simulink model "M_DYN_AerodynamicData"  (R2022a)
settings: Solver=ode4  StartTime=0.0  StopTime=0.04  FixedStep=0.01  RelTol=1e-3
PreLoadFcn:
  | load('f16data.mat');
InitFcn:
  | load('f16data.mat');
values from neighbouring files (symbols this model uses):
  f16data =     [f16data.mat]
settings Model: Creator=ASCL  LastModifiedBy=ASCL
settings DataIOCC: SaveOutput=off  SignalLogging=off  DSMLogging=off  SaveTime=off  ReturnWorkspaceOutputs=off
settings OptimizationCC: BlockReduction=off  DefaultParameterBehavior=Inlined  UseDivisionForNetSlopeComputation=on  GainParamInheritBuiltInType=on  UseFloatMulNetSlope=on  ExpressionFolding=off  PassReuseOutputArgsAs=Individual arguments  ZeroExternalMemoryAtStartup=off  ZeroInternalMemoryAtStartup=off  EfficientFloat2IntCast=on  LifeSpan=inf  OptimizeBlockOrder=speed  DifferentSizesBufferReuse=on  EfficientTunableParamExpr=on
settings DebuggingCC: SignalInfNanChecking=warning  ReadBeforeWriteMsg=EnableAllAsError  WriteAfterWriteMsg=EnableAllAsError  WriteAfterReadMsg=EnableAllAsError  IntegerOverflowMsg=error  ParameterTunabilityLossMsg=error  UniqueDataStoreMsg=error  AssertControl=DisableAll  NonBusSignalsTreatedAsBus=error  SFInvalidInputDataAccessInChartInitDiag=error  SFTransitionOutsideNaturalParentDiag=error  SFUnreachableExecutionPathDiag=error  SFUndirectedBroadcastEventsDiag=error  IntegerSaturationMsg=error
settings HardwareCC: ProdBitPerPointer=32  ProdBitPerSizeT=32  ProdBitPerPtrDiffT=32  ProdLargestAtomicInteger=Long  ProdLargestAtomicFloat=Double  ProdEndianess=BigEndian  ProdWordSize=32  ProdLongLongMode=on  ProdHWDeviceType=Freescale->MPC83xx
settings SFSimCC: CompileTimeRecursionLimit=0  EnableRuntimeRecursion=off  MATLABDynamicMemAlloc=off
settings RTWCC: SystemTargetFile=ert.tlc  TemplateMakefile=ert_default_tmf  GenerateReport=on  RTWUseSimCustomCode=on  BuildConfiguration=Faster Runs  IncludeHyperlinkInReport=on  LaunchReport=on  GenerateTraceInfo=on  GenerateTraceReport=on  GenerateTraceReportSl=on  GenerateTraceReportSf=on  GenerateTraceReportEml=on
settings CodeAppCC: ForceParamTrailComments=on  IgnoreCustomStorageClasses=off  OperatorAnnotations=on  SimulinkDataObjDesc=on  SFDataObjDesc=on  MATLABFcnDesc=on  InsertBlockDesc=on  StateflowObjectComments=on  MATLABSourceComments=on  EnableCustomComments=on  InlinedPrmAccess=Macros  ReqsInCode=on
settings ERTTargetCC: TargetLangStandard=C99 (ISO)  UtilityFuncGeneration=Shared location  GenerateSampleERTMain=on  IncludeMdlTerminateFcn=off  CombineSignalStateStructs=on  SupportAbsoluteTime=off  SupportNonFinite=off  SupportVariableSizeSignals=on  ParenthesesLevel=Standards  CastingMode=Standards  GenerateSharedConstants=off  InlinedParameterPlacement=NonHierarchical  ERTCustomFileTemplate=example_file_process.tlc  RateTransitionBlockCode=Function  PreserveIfCondition=on  ConvertIfToSwitch=off  EnableSignedLeftShifts=off  EnableSignedRightShifts=off

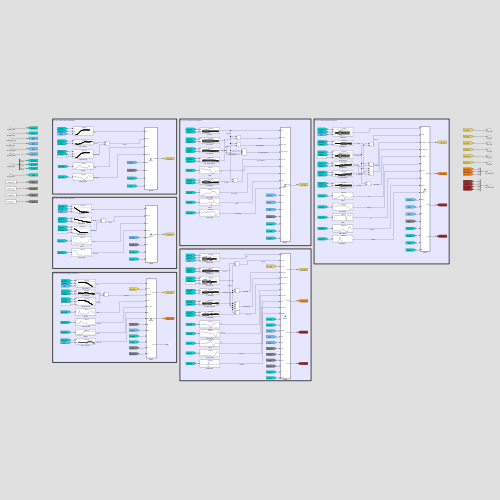
[thumbnail: Simulink's stored preview of the top-level diagram]
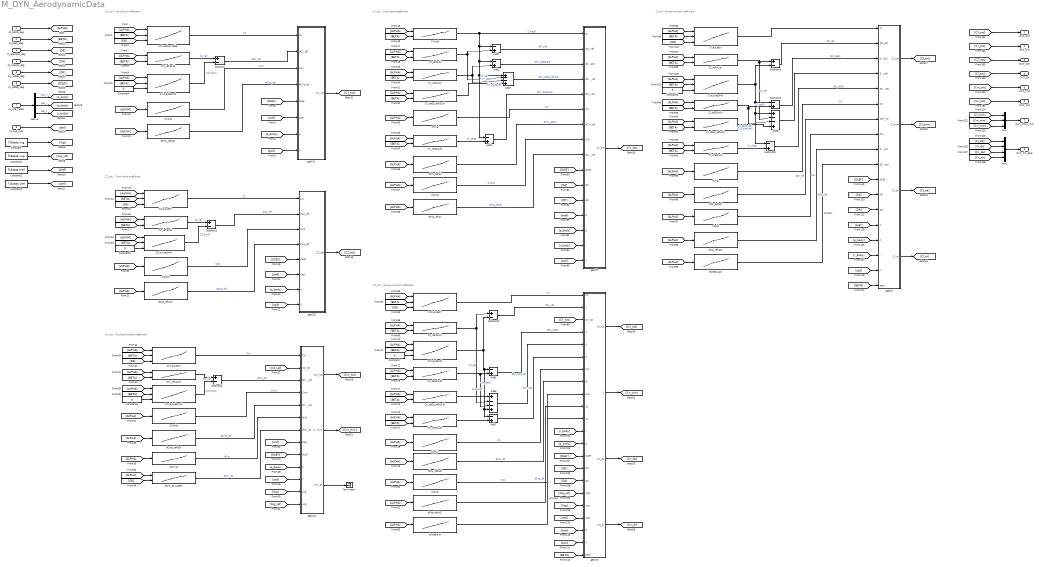
== system M_DYN_AerodynamicData ==
  note: Cl_tot : rolling moment coefficient
  note: Cn_tot : yawing moment coefficient
  note: CY_tot : Y-axis force coefficient
  note: Cm_tot : Pitching moment coefficient
  note: CZ_tot : Z-axis force coefficient
  note: CX_tot: X-axis force coefficient
  IN_alpha_deg : Inport  Interpolate=off
  IN_beta_deg : Inport  Port=2  Interpolate=off
  IN_elevator_deg : Inport  Port=3  Interpolate=off
  IN_aileron_deg : Inport  Port=4  Interpolate=off
  IN_rudder_deg : Inport  Port=5  Interpolate=off
  IN_LEflap_deg : Inport  Port=6  Interpolate=off
  IN_WB_radps : Inport  Port=7  Interpolate=off
  IN_spd_mps : Inport  Port=8  Interpolate=off
  Add{1..2,4..5,7} (5 alike) : Sum  Inputs=-+
  Add3 : Sum  Inputs=+--+
  Add6 : Sum  Inputs=+--+
  Add8 : Sum  Inputs=+--+
  CX(a,b,de1=0) : Lookup_n-D  NumberOfTableDimensions=3  BreakpointsForDimension1=f16data.alpha1  BreakpointsForDimension2=f16data.beta  BreakpointsForDimension3=f16data.de1  Table=f16data.CX  InternalRulePriority=Speed  RndMeth=Simplest
      settings: InputPortMap=u0,u1,u2
  CX_lef(a2,b) : Lookup_n-D  LookupTableObject=''  BreakpointsForDimension1=f16data.alpha2  BreakpointsForDimension2=f16data.beta  BreakpointsForDimension1FirstPoint=10  BreakpointsForDimension2FirstPoint=10  BreakpointsForDimension1Spacing=12  BreakpointsForDimension2Spacing=12  Table=f16data.CX_lef  DiagnosticForOutOfRangeInput=Warning  InternalRulePriority=Speed  RndMeth=Simplest
      settings: InputPortMap=u0,u1
  CXq(a) : Lookup_n-D  NumberOfTableDimensions=1  BreakpointsForDimension1=f16data.alpha1  Table=f16data.CXq  InternalRulePriority=Speed  RndMeth=Simplest
  CY(a,b) : Lookup_n-D  LookupTableObject=''  BreakpointsForDimension1=f16data.alpha1  BreakpointsForDimension2=f16data.beta  BreakpointsForDimension1FirstPoint=10  BreakpointsForDimension2FirstPoint=10  BreakpointsForDimension1Spacing=12  BreakpointsForDimension2Spacing=12  Table=f16data.CY  DiagnosticForOutOfRangeInput=Warning  InternalRulePriority=Speed  RndMeth=Simplest
      settings: InputPortMap=u0,u1
  CY_a20(a,b) : Lookup_n-D  LookupTableObject=''  BreakpointsForDimension1=f16data.alpha1  BreakpointsForDimension2=f16data.beta  BreakpointsForDimension1FirstPoint=10  BreakpointsForDimension2FirstPoint=10  BreakpointsForDimension1Spacing=12  BreakpointsForDimension2Spacing=12  Table=f16data.CY_da20  DiagnosticForOutOfRangeInput=Warning  InternalRulePriority=Speed  RndMeth=Simplest
      settings: InputPortMap=u0,u1
  CY_da20_lef(a2,b) : Lookup_n-D  LookupTableObject=''  BreakpointsForDimension1=f16data.alpha2  BreakpointsForDimension2=f16data.beta  BreakpointsForDimension1FirstPoint=10  BreakpointsForDimension2FirstPoint=10  BreakpointsForDimension1Spacing=12  BreakpointsForDimension2Spacing=12  Table=f16data.CY_da20lef  DiagnosticForOutOfRangeInput=Warning  InternalRulePriority=Speed  RndMeth=Simplest
      settings: InputPortMap=u0,u1
  CY_dr30(a,b) : Lookup_n-D  LookupTableObject=''  BreakpointsForDimension1=f16data.alpha1  BreakpointsForDimension2=f16data.beta  BreakpointsForDimension1FirstPoint=10  BreakpointsForDimension2FirstPoint=10  BreakpointsForDimension1Spacing=12  BreakpointsForDimension2Spacing=12  Table=f16data.CY_dr30  DiagnosticForOutOfRangeInput=Warning  InternalRulePriority=Speed  RndMeth=Simplest
      settings: InputPortMap=u0,u1
  CY_lef(a,b) : Lookup_n-D  LookupTableObject=''  BreakpointsForDimension1=f16data.alpha2  BreakpointsForDimension2=f16data.beta  BreakpointsForDimension1FirstPoint=10  BreakpointsForDimension2FirstPoint=10  BreakpointsForDimension1Spacing=12  BreakpointsForDimension2Spacing=12  Table=f16data.CY_lef  DiagnosticForOutOfRangeInput=Warning  InternalRulePriority=Speed  RndMeth=Simplest
      settings: InputPortMap=u0,u1
  CYp(a) : Lookup_n-D  NumberOfTableDimensions=1  LookupTableObject=''  BreakpointsForDimension1=f16data.alpha1  BreakpointsForDimension2=f16data.beta  BreakpointsForDimension1FirstPoint=10  BreakpointsForDimension2FirstPoint=10  BreakpointsForDimension1Spacing=12  BreakpointsForDimension2Spacing=12  Table=f16data.CYp  DiagnosticForOutOfRangeInput=Warning  InternalRulePriority=Speed  RndMeth=Simplest
  CYr(a) : Lookup_n-D  NumberOfTableDimensions=1  LookupTableObject=''  BreakpointsForDimension1=f16data.alpha1  BreakpointsForDimension2=f16data.beta  BreakpointsForDimension1FirstPoint=10  BreakpointsForDimension2FirstPoint=10  BreakpointsForDimension1Spacing=12  BreakpointsForDimension2Spacing=12  Table=f16data.CYr  DiagnosticForOutOfRangeInput=Warning  InternalRulePriority=Speed  RndMeth=Simplest
  CZ(a,b,de1) : Lookup_n-D  NumberOfTableDimensions=3  BreakpointsForDimension1=f16data.alpha1  BreakpointsForDimension2=f16data.beta  BreakpointsForDimension3=f16data.de1  BeginIndexSearchUsingPreviousIndexResult=on  Table=f16data.CZ  InternalRulePriority=Speed  RndMeth=Simplest
      settings: InputPortMap=u0,u1,u2
  CZ(a,b,de1=0) : Lookup_n-D  NumberOfTableDimensions=3  BreakpointsForDimension1=f16data.alpha1  BreakpointsForDimension2=f16data.beta  BreakpointsForDimension3=f16data.de1  BeginIndexSearchUsingPreviousIndexResult=on  Table=f16data.CZ  InternalRulePriority=Speed  RndMeth=Simplest
      settings: InputPortMap=u0,u1,u2
  CZ_lef(a2,b) : Lookup_n-D  LookupTableObject=''  BreakpointsForDimension1=f16data.alpha2  BreakpointsForDimension2=f16data.beta  BreakpointsForDimension1FirstPoint=10  BreakpointsForDimension2FirstPoint=10  BreakpointsForDimension1Spacing=12  BreakpointsForDimension2Spacing=12  BeginIndexSearchUsingPreviousIndexResult=on  Table=f16data.CZ_lef  DiagnosticForOutOfRangeInput=Warning  InternalRulePriority=Speed  RndMeth=Simplest
      settings: InputPortMap=u0,u1
  CZq(a) : Lookup_n-D  NumberOfTableDimensions=1  BreakpointsForDimension1=f16data.alpha1  BeginIndexSearchUsingPreviousIndexResult=on  Table=f16data.CZq  InternalRulePriority=Speed  RndMeth=Simplest
  Cl(a,b,de2) : Lookup_n-D  NumberOfTableDimensions=3  BreakpointsForDimension1=f16data.alpha1  BreakpointsForDimension2=f16data.beta  BreakpointsForDimension3=f16data.de2  Table=f16data.Cl  InternalRulePriority=Speed  RndMeth=Simplest
      settings: InputPortMap=u0,u1,u2
  Cl(a,b,de2=0) : Lookup_n-D  NumberOfTableDimensions=3  BreakpointsForDimension1=f16data.alpha1  BreakpointsForDimension2=f16data.beta  BreakpointsForDimension3=f16data.de2  Table=f16data.Cl  InternalRulePriority=Speed  RndMeth=Simplest
      settings: InputPortMap=u0,u1,u2
  Cl_da20(a,b) : Lookup_n-D  LookupTableObject=''  BreakpointsForDimension1=f16data.alpha1  BreakpointsForDimension2=f16data.beta  BreakpointsForDimension1FirstPoint=10  BreakpointsForDimension2FirstPoint=10  BreakpointsForDimension1Spacing=12  BreakpointsForDimension2Spacing=12  Table=f16data.Cl_da20  DiagnosticForOutOfRangeInput=Warning  InternalRulePriority=Speed  RndMeth=Simplest
      settings: InputPortMap=u0,u1
  Cl_da20_lef(a,b) : Lookup_n-D  LookupTableObject=''  BreakpointsForDimension1=f16data.alpha2  BreakpointsForDimension2=f16data.beta  BreakpointsForDimension1FirstPoint=10  BreakpointsForDimension2FirstPoint=10  BreakpointsForDimension1Spacing=12  BreakpointsForDimension2Spacing=12  Table=f16data.Cl_da20lef  DiagnosticForOutOfRangeInput=Warning  InternalRulePriority=Speed  RndMeth=Simplest
      settings: InputPortMap=u0,u1
  Cl_dr30(a,b) : Lookup_n-D  LookupTableObject=''  BreakpointsForDimension1=f16data.alpha1  BreakpointsForDimension2=f16data.beta  BreakpointsForDimension1FirstPoint=10  BreakpointsForDimension2FirstPoint=10  BreakpointsForDimension1Spacing=12  BreakpointsForDimension2Spacing=12  Table=f16data.Cl_dr30  DiagnosticForOutOfRangeInput=Warning  InternalRulePriority=Speed  RndMeth=Simplest
      settings: InputPortMap=u0,u1
  Cl_lef(a2,b) : Lookup_n-D  LookupTableObject=''  BreakpointsForDimension1=f16data.alpha2  BreakpointsForDimension2=f16data.beta  BreakpointsForDimension1FirstPoint=10  BreakpointsForDimension2FirstPoint=10  BreakpointsForDimension1Spacing=12  BreakpointsForDimension2Spacing=12  Table=f16data.Cl_lef  DiagnosticForOutOfRangeInput=Warning  InternalRulePriority=Speed  RndMeth=Simplest
      settings: InputPortMap=u0,u1
  Clp(a) : Lookup_n-D  NumberOfTableDimensions=1  LookupTableObject=''  BreakpointsForDimension1=f16data.alpha1  BreakpointsForDimension2=f16data.beta  BreakpointsForDimension1FirstPoint=10  BreakpointsForDimension2FirstPoint=10  BreakpointsForDimension1Spacing=12  BreakpointsForDimension2Spacing=12  Table=f16data.Clp  DiagnosticForOutOfRangeInput=Warning  InternalRulePriority=Speed  RndMeth=Simplest
  Clr(a) : Lookup_n-D  NumberOfTableDimensions=1  LookupTableObject=''  BreakpointsForDimension1=f16data.alpha1  BreakpointsForDimension2=f16data.beta  BreakpointsForDimension1FirstPoint=10  BreakpointsForDimension2FirstPoint=10  BreakpointsForDimension1Spacing=12  BreakpointsForDimension2Spacing=12  Table=f16data.Clr  DiagnosticForOutOfRangeInput=Warning  InternalRulePriority=Speed  RndMeth=Simplest
  Cm(a,b,de1) : Lookup_n-D  NumberOfTableDimensions=3  BreakpointsForDimension1=f16data.alpha1  BreakpointsForDimension2=f16data.beta  BreakpointsForDimension3=f16data.de1  Table=f16data.Cm  InternalRulePriority=Speed  RndMeth=Simplest
      settings: InputPortMap=u0,u1,u2
  Cm(a,b,de1=0) : Lookup_n-D  NumberOfTableDimensions=3  BreakpointsForDimension1=f16data.alpha1  BreakpointsForDimension2=f16data.beta  BreakpointsForDimension3=f16data.de1  Table=f16data.Cm  InternalRulePriority=Speed  RndMeth=Simplest
      settings: InputPortMap=u0,u1,u2
  Cm_lef(a2,b) : Lookup_n-D  LookupTableObject=''  BreakpointsForDimension1=f16data.alpha2  BreakpointsForDimension2=f16data.beta  BreakpointsForDimension1FirstPoint=10  BreakpointsForDimension2FirstPoint=10  BreakpointsForDimension1Spacing=12  BreakpointsForDimension2Spacing=12  Table=f16data.Cm_lef  DiagnosticForOutOfRangeInput=Warning  InternalRulePriority=Speed  RndMeth=Simplest
      settings: InputPortMap=u0,u1
  Cmq(a) : Lookup_n-D  NumberOfTableDimensions=1  BreakpointsForDimension1=f16data.alpha1  Table=f16data.Cmq  InternalRulePriority=Speed  RndMeth=Simplest
  Cn(a,b,de2) : Lookup_n-D  NumberOfTableDimensions=3  BreakpointsForDimension1=f16data.alpha1  BreakpointsForDimension2=f16data.beta  BreakpointsForDimension3=f16data.de2  Table=f16data.Cn  InternalRulePriority=Speed  RndMeth=Simplest
      settings: InputPortMap=u0,u1,u2
  Cn(a,b,de=0) : Lookup_n-D  NumberOfTableDimensions=3  BreakpointsForDimension1=f16data.alpha1  BreakpointsForDimension2=f16data.beta  BreakpointsForDimension3=f16data.de2  Table=f16data.Cn  InternalRulePriority=Speed  RndMeth=Simplest
      settings: InputPortMap=u0,u1,u2
  Cn_da20(a,b) : Lookup_n-D  LookupTableObject=''  BreakpointsForDimension1=f16data.alpha1  BreakpointsForDimension2=f16data.beta  BreakpointsForDimension1FirstPoint=10  BreakpointsForDimension2FirstPoint=10  BreakpointsForDimension1Spacing=12  BreakpointsForDimension2Spacing=12  Table=f16data.Cn_da20  DiagnosticForOutOfRangeInput=Warning  InternalRulePriority=Speed  RndMeth=Simplest
      settings: InputPortMap=u0,u1
  Cn_da20_lef(a2,b) : Lookup_n-D  LookupTableObject=''  BreakpointsForDimension1=f16data.alpha2  BreakpointsForDimension2=f16data.beta  BreakpointsForDimension1FirstPoint=10  BreakpointsForDimension2FirstPoint=10  BreakpointsForDimension1Spacing=12  BreakpointsForDimension2Spacing=12  Table=f16data.Cn_da20lef  DiagnosticForOutOfRangeInput=Warning  InternalRulePriority=Speed  RndMeth=Simplest
      settings: InputPortMap=u0,u1
  Cn_dr30(a,b) : Lookup_n-D  LookupTableObject=''  BreakpointsForDimension1=f16data.alpha1  BreakpointsForDimension2=f16data.beta  BreakpointsForDimension1FirstPoint=10  BreakpointsForDimension2FirstPoint=10  BreakpointsForDimension1Spacing=12  BreakpointsForDimension2Spacing=12  Table=f16data.Cn_dr30  DiagnosticForOutOfRangeInput=Warning  InternalRulePriority=Speed  RndMeth=Simplest
      settings: InputPortMap=u0,u1
  Cn_lef(a2,b) : Lookup_n-D  LookupTableObject=''  BreakpointsForDimension1=f16data.alpha2  BreakpointsForDimension2=f16data.beta  BreakpointsForDimension1FirstPoint=10  BreakpointsForDimension2FirstPoint=10  BreakpointsForDimension1Spacing=12  BreakpointsForDimension2Spacing=12  Table=f16data.Cn_lef  DiagnosticForOutOfRangeInput=Warning  InternalRulePriority=Speed  RndMeth=Simplest
      settings: InputPortMap=u0,u1
  Cnp(a) : Lookup_n-D  NumberOfTableDimensions=1  LookupTableObject=''  BreakpointsForDimension1=f16data.alpha1  BreakpointsForDimension2=f16data.beta  BreakpointsForDimension1FirstPoint=10  BreakpointsForDimension2FirstPoint=10  BreakpointsForDimension1Spacing=12  BreakpointsForDimension2Spacing=12  Table=f16data.Cnp  DiagnosticForOutOfRangeInput=Warning  InternalRulePriority=Speed  RndMeth=Simplest
  Cnr(a) : Lookup_n-D  NumberOfTableDimensions=1  LookupTableObject=''  BreakpointsForDimension1=f16data.alpha1  BreakpointsForDimension2=f16data.beta  BreakpointsForDimension1FirstPoint=10  BreakpointsForDimension2FirstPoint=10  BreakpointsForDimension1Spacing=12  BreakpointsForDimension2Spacing=12  Table=f16data.Cnr  DiagnosticForOutOfRangeInput=Warning  InternalRulePriority=Speed  RndMeth=Simplest
  Constant : Constant  Value=f16data.xcg
  Constant1 : Constant  Value=f16data.xcgr
  Constant2 : Constant  Value=f16data.bref
  Constant3 : Constant  Value=f16data.cref
  Constant{4..8} (5 alike) : Constant  Value=0
  Demux : Demux  Outputs=3
  Mux : Mux  Inputs=3
  Mux1 : Mux
  Subtract{,1..4} (5 alike) : Sum  Inputs=+-
  Subtract5 : Sum  Inputs=-+
  Subtract6 : Sum  Inputs=-+
  Terminator : Terminator
  dCXq_lef(a2) : Lookup_n-D  NumberOfTableDimensions=1  BreakpointsForDimension1=f16data.alpha2  Table=f16data.dCXq_lef  InternalRulePriority=Speed  RndMeth=Simplest
  dCYp_lef(a) : Lookup_n-D  NumberOfTableDimensions=1  LookupTableObject=''  BreakpointsForDimension1=f16data.alpha2  BreakpointsForDimension2=f16data.beta  BreakpointsForDimension1FirstPoint=10  BreakpointsForDimension2FirstPoint=10  BreakpointsForDimension1Spacing=12  BreakpointsForDimension2Spacing=12  Table=f16data.dCYp_lef  DiagnosticForOutOfRangeInput=Warning  InternalRulePriority=Speed  RndMeth=Simplest
  dCYr_lef(a) : Lookup_n-D  NumberOfTableDimensions=1  LookupTableObject=''  BreakpointsForDimension1=f16data.alpha2  BreakpointsForDimension2=f16data.beta  BreakpointsForDimension1FirstPoint=10  BreakpointsForDimension2FirstPoint=10  BreakpointsForDimension1Spacing=12  BreakpointsForDimension2Spacing=12  Table=f16data.dCYr_lef  DiagnosticForOutOfRangeInput=Warning  InternalRulePriority=Speed  RndMeth=Simplest
  dCZq_lef(a2) : Lookup_n-D  NumberOfTableDimensions=1  BreakpointsForDimension1=f16data.alpha2  BeginIndexSearchUsingPreviousIndexResult=on  Table=f16data.dCZq_lef  InternalRulePriority=Speed  RndMeth=Simplest
  dClbeta(a1) : Lookup_n-D  NumberOfTableDimensions=1  LookupTableObject=''  BreakpointsForDimension1=f16data.alpha1  BreakpointsForDimension2=f16data.beta  BreakpointsForDimension1FirstPoint=10  BreakpointsForDimension2FirstPoint=10  BreakpointsForDimension1Spacing=12  BreakpointsForDimension2Spacing=12  Table=f16data.dClbeta  DiagnosticForOutOfRangeInput=Warning  InternalRulePriority=Speed  RndMeth=Simplest
  dClp_lef(a2) : Lookup_n-D  NumberOfTableDimensions=1  LookupTableObject=''  BreakpointsForDimension1=f16data.alpha2  BreakpointsForDimension2=f16data.beta  BreakpointsForDimension1FirstPoint=10  BreakpointsForDimension2FirstPoint=10  BreakpointsForDimension1Spacing=12  BreakpointsForDimension2Spacing=12  Table=f16data.dClp_lef  DiagnosticForOutOfRangeInput=Warning  InternalRulePriority=Speed  RndMeth=Simplest
  dClr_lef(a2) : Lookup_n-D  NumberOfTableDimensions=1  LookupTableObject=''  BreakpointsForDimension1=f16data.alpha2  BreakpointsForDimension2=f16data.beta  BreakpointsForDimension1FirstPoint=10  BreakpointsForDimension2FirstPoint=10  BreakpointsForDimension1Spacing=12  BreakpointsForDimension2Spacing=12  Table=f16data.dClr_lef  DiagnosticForOutOfRangeInput=Warning  InternalRulePriority=Speed  RndMeth=Simplest
  dCm(a) : Lookup_n-D  NumberOfTableDimensions=1  BreakpointsForDimension1=f16data.alpha1  Table=f16data.dCm  InternalRulePriority=Speed  RndMeth=Simplest
  dCm_ds(a,de3) : Lookup_n-D  LookupTableObject=''  BreakpointsForDimension1=f16data.alpha1  BreakpointsForDimension2=f16data.de3  BreakpointsForDimension1FirstPoint=10  BreakpointsForDimension2FirstPoint=10  BreakpointsForDimension1Spacing=12  BreakpointsForDimension2Spacing=12  Table=f16data.dCm_ds  DiagnosticForOutOfRangeInput=Warning  InternalRulePriority=Speed  RndMeth=Simplest
      settings: InputPortMap=u0,u1
  dCmq_lef(a2) : Lookup_n-D  NumberOfTableDimensions=1  BreakpointsForDimension1=f16data.alpha2  Table=f16data.dCmq_lef  InternalRulePriority=Speed  RndMeth=Simplest
  dCnbeta(a) : Lookup_n-D  NumberOfTableDimensions=1  LookupTableObject=''  BreakpointsForDimension1=f16data.alpha1  BreakpointsForDimension2=f16data.beta  BreakpointsForDimension1FirstPoint=10  BreakpointsForDimension2FirstPoint=10  BreakpointsForDimension1Spacing=12  BreakpointsForDimension2Spacing=12  Table=f16data.dCnbeta  DiagnosticForOutOfRangeInput=Warning  InternalRulePriority=Speed  RndMeth=Simplest
  dCnp_lef(a2) : Lookup_n-D  NumberOfTableDimensions=1  LookupTableObject=''  BreakpointsForDimension1=f16data.alpha2  BreakpointsForDimension2=f16data.beta  BreakpointsForDimension1FirstPoint=10  BreakpointsForDimension2FirstPoint=10  BreakpointsForDimension1Spacing=12  BreakpointsForDimension2Spacing=12  Table=f16data.dCnp_lef  DiagnosticForOutOfRangeInput=Warning  InternalRulePriority=Speed  RndMeth=Simplest
  dCnr_lef(a2) : Lookup_n-D  NumberOfTableDimensions=1  LookupTableObject=''  BreakpointsForDimension1=f16data.alpha2  BreakpointsForDimension2=f16data.beta  BreakpointsForDimension1FirstPoint=10  BreakpointsForDimension2FirstPoint=10  BreakpointsForDimension1Spacing=12  BreakpointsForDimension2Spacing=12  Table=f16data.dCnr_lef  DiagnosticForOutOfRangeInput=Warning  InternalRulePriority=Speed  RndMeth=Simplest
  getCXt : MATLAB Function  TreatAsAtomicUnit=on
  getCYt : MATLAB Function  TreatAsAtomicUnit=on
  getCZt : MATLAB Function  TreatAsAtomicUnit=on
  getClt : MATLAB Function  TreatAsAtomicUnit=on
  getCmt : MATLAB Function  TreatAsAtomicUnit=on
  getCnt : MATLAB Function  TreatAsAtomicUnit=on
  n-D Lookup Table : Lookup_n-D  NumberOfTableDimensions=3  BreakpointsForDimension1=f16data.alpha1  BreakpointsForDimension2=f16data.beta  BreakpointsForDimension3=f16data.de1  Table=f16data.CX  InternalRulePriority=Speed  RndMeth=Simplest
      settings: InputPortMap=u0,u1,u2
  OUT_CXt : Outport  VectorParamsAs1DForOutWhenUnconnected=off
  OUT_CYt : Outport  Port=2  VectorParamsAs1DForOutWhenUnconnected=off
  OUT_CZt : Outport  Port=3  VectorParamsAs1DForOutWhenUnconnected=off
  OUT_Clt : Outport  Port=4  VectorParamsAs1DForOutWhenUnconnected=off
  OUT_Cmt : Outport  Port=5  VectorParamsAs1DForOutWhenUnconnected=off
  OUT_Cnt : Outport  Port=6  VectorParamsAs1DForOutWhenUnconnected=off
  OUT_Clmn_trim : Outport  Port=7
  OUT_Cln_dadr : Outport  Port=8
  wires:
  IN_alpha_deg/1 -> [ALPHA]
  IN_beta_deg/1 -> [BETA]
  IN_elevator_deg/1 -> [DE]
  IN_aileron_deg/1 -> [DA]
  IN_rudder_deg/1 -> [DR]
  IN_LEflap_deg/1 -> [DLEF]
  IN_WB_radps/1 -> Demux/1
  Demux/1 -> [p_body]  "WB_x"
  Demux/2 -> [q_body]  "WB_y"
  Demux/3 -> [r_body]  "WB_z"
  IN_spd_mps/1 -> [spd]
  Constant/1 -> [Xcg]
  Constant1/1 -> [Xcg_ref]
  Constant2/1 -> [bref]
  Constant3/1 -> [cref]
  [ALPHA] -> n-D Lookup Table/1
  [BETA] -> n-D Lookup Table/2
  [DE] -> n-D Lookup Table/3
  n-D Lookup Table/1 -> getCXt/1(CX)  "CX"
  getCXt/1(CX_tot) -> [CX_tot]
  [spd] -> getCXt/8(V)
  [q_body] -> getCXt/7(q)
  [cref] -> getCXt/6(cbar)
  [DLEF] -> getCXt/5(DLEF)
  CXq(a)/1 -> getCXt/3(CXq)  "CXq"
  dCXq_lef(a2)/1 -> getCXt/4(dCXq_lef)  "dCXq_lef"
  CX_lef(a2,b)/1 -> Subtract/1  "CX_lef"
  CX(a,b,de1=0)/1 -> Subtract/2  "CX(a,b,0)"
  Subtract/1 -> getCXt/2(dCX_lef)  "dCX_lef"
  [ALPHA] -> CX_lef(a2,b)/1
  [BETA] -> CX_lef(a2,b)/2
  [BETA] -> CX(a,b,de1=0)/2
  [ALPHA] -> CX(a,b,de1=0)/1
  Constant4/1 -> CX(a,b,de1=0)/3
  [ALPHA] -> dCXq_lef(a2)/1
  [ALPHA] -> CXq(a)/1
  [ALPHA] -> CZ(a,b,de1)/1
  [BETA] -> CZ(a,b,de1)/2
  [DE] -> CZ(a,b,de1)/3
  [ALPHA] -> CZ_lef(a2,b)/1
  [BETA] -> CZ_lef(a2,b)/2
  [ALPHA] -> CZ(a,b,de1=0)/1
  [BETA] -> CZ(a,b,de1=0)/2
  Constant5/1 -> CZ(a,b,de1=0)/3
  [ALPHA] -> dCZq_lef(a2)/1
  [ALPHA] -> CZq(a)/1
  [DLEF] -> getCZt/5(DLEF)
  [spd] -> getCZt/8(V)
  [q_body] -> getCZt/7(q)
  [cref] -> getCZt/6(cbar)
  dCZq_lef(a2)/1 -> getCZt/4(CZq_lef)  "dCZq_lef"
  CZq(a)/1 -> getCZt/3(CZq)  "CZq"
  CZ(a,b,de1)/1 -> getCZt/1(CZ)  "CZ"
  CZ_lef(a2,b)/1 -> Subtract1/1  "CZ_lef"
  CZ(a,b,de1=0)/1 -> Subtract1/2  "CZ(a,b,0)"
  Subtract1/1 -> getCZt/2(dCZ_lef)  "dCZ_lef"
  getCZt/1(CZ_tot) -> [CZ_tot]
  getCmt/1(Cm_tot) -> [Cm_tot]
  getCmt/2(Cm_trim) -> [Cm_trim]
  getCmt/3(Cm_de) -> Terminator/1
  [cref] -> getCmt/8(cbar)
  [DLEF] -> getCmt/9(DLEF)
  [q_body] -> getCmt/10(q)
  [spd] -> getCmt/11(V)
  [Xcg] -> getCmt/12(xcg)
  [Xcg_ref] -> getCmt/13(xcgr)
  [CZ_tot] -> getCmt/2(CZ_tot)
  [ALPHA] -> dCm_ds(a,de3)/1
  [DE] -> dCm_ds(a,de3)/2
  dCm_ds(a,de3)/1 -> getCmt/7(dCm_ds)  "dCm_ds"
  [ALPHA] -> dCm(a)/1
  [ALPHA] -> dCmq_lef(a2)/1
  dCmq_lef(a2)/1 -> getCmt/5(dCmq_lef)  "dCmq_lef"
  dCm(a)/1 -> getCmt/6(dCm)  "dCm"
  [ALPHA] -> Cmq(a)/1
  Cmq(a)/1 -> getCmt/4(Cmq)  "Cmq"
  Constant6/1 -> Cm(a,b,de1=0)/3
  [BETA] -> Cm(a,b,de1=0)/2
  [ALPHA] -> Cm(a,b,de1=0)/1
  [BETA] -> Cm_lef(a2,b)/2
  [ALPHA] -> Cm_lef(a2,b)/1
  [DE] -> Cm(a,b,de1)/3
  [BETA] -> Cm(a,b,de1)/2
  [ALPHA] -> Cm(a,b,de1)/1
  Cm(a,b,de1)/1 -> getCmt/1(Cm)  "Cm"
  Cm_lef(a2,b)/1 -> Subtract2/1  "Cm_lef"
  Cm(a,b,de1=0)/1 -> Subtract2/2  "Cm(a,b,0)"
  Subtract2/1 -> getCmt/3(dCm_lef)  "dCm_lef"
  dCYp_lef(a)/1 -> getCYt/9(dCYp_lef)  "dCYp_lef(a)"
  CYr(a)/1 -> getCYt/6(CYr)  "CYr"
  dCYr_lef(a)/1 -> getCYt/7(dCYr_lef)  "dCYr_lef(a)"
  CYp(a)/1 -> getCYt/8(CYp)  "CYp(a)"
  CY_da20_lef(a2,b)/1 -> Add3/4  "CY_da20_lef"
  CY_dr30(a,b)/1 -> Add4/2  "CY_dr30"
  CY_a20(a,b)/1 -> Add3/3, Add2/2  "CY_da20"
  Add2/1 -> getCYt/3(dCY_a20)  "dCY_da20(a,b)"
  Add4/1 -> getCYt/5(dCY_r30)  "dCY_dr30(a,b)"
  Add3/1 -> getCYt/4(dCY_a20_lef)  "dCY_da20_lef(a,b)"
  Add1/1 -> getCYt/2(dCY_lef)  "dCY_lef"
  CY_lef(a,b)/1 -> Add3/2, Add1/2  "CY_lef"
  CY(a,b)/1 -> Add4/1, Add3/1, Add2/1, Add1/1, getCYt/1(CY)  "CY(a,b)"
  [BETA] -> CY(a,b)/2
  [BETA] -> CY_lef(a,b)/2
  [BETA] -> CY_dr30(a,b)/2
  [ALPHA] -> dCYr_lef(a)/1
  [ALPHA] -> dCYp_lef(a)/1
  [ALPHA] -> CY(a,b)/1
  [ALPHA] -> CY_lef(a,b)/1
  [BETA] -> CY_a20(a,b)/2
  [ALPHA] -> CY_a20(a,b)/1
  [BETA] -> CY_da20_lef(a2,b)/2
  [ALPHA] -> CY_da20_lef(a2,b)/1
  [ALPHA] -> CYr(a)/1
  [ALPHA] -> CY_dr30(a,b)/1
  [ALPHA] -> CYp(a)/1
  [bref] -> getCYt/13(b)
  [DLEF] -> getCYt/10(DLEF)
  [DR] -> getCYt/12(DR)
  [DA] -> getCYt/11(DA)
  [p_body] -> getCYt/14(p)
  [r_body] -> getCYt/15(r)
  [spd] -> getCYt/16(V)
  getCYt/1(CY_tot) -> [CY_tot]
  dCnr_lef(a2)/1 -> getCnt/8(dCnr_lef)  "dCnr_lef"
  dCnbeta(a)/1 -> getCnt/11(dCnbeta)  "dCnbeta"
  Add5/1 -> getCnt/4(dCn_a20)  "dCn_da20"
  Add6/1 -> getCnt/5(dCn_a20_lef)  "dCn_a20_lef"
  Cn_da20_lef(a2,b)/1 -> Add6/1
  Cn(a,b,de=0)/1 -> Add7/1, Add6/4, Add5/1, Subtract3/2  "Cn(a,b,0)"
  Subtract3/1 -> getCnt/2(dCn_lef)  "dCn_lef"
  dCnp_lef(a2)/1 -> getCnt/10(dCnp_lef)  "dCnp_lef"
  Cnr(a)/1 -> getCnt/7(Cnr)  "Cnr"
  Cn_da20(a,b)/1 -> Add6/3, Add5/2  "Cn_da20"
  Cn_lef(a2,b)/1 -> Add6/2, Subtract3/1  "Cn_lef"
  Cn(a,b,de2)/1 -> getCnt/1(Cn)  "Cn"
  Cn_dr30(a,b)/1 -> Add7/2
  Cnp(a)/1 -> getCnt/9(Cnp)  "Cnp"
  Add7/1 -> getCnt/6(dCn_r30)  "dCn_r30"
  [BETA] -> Cn(a,b,de2)/2
  [ALPHA] -> Cn(a,b,de2)/1
  [BETA] -> Cn_lef(a2,b)/2
  [BETA] -> Cn(a,b,de=0)/2
  [BETA] -> Cn_da20(a,b)/2
  [BETA] -> Cn_da20_lef(a2,b)/2
  [ALPHA] -> Cnr(a)/1
  [ALPHA] -> Cnp(a)/1
  [ALPHA] -> dCnbeta(a)/1
  [ALPHA] -> dCnp_lef(a2)/1
  [ALPHA] -> dCnr_lef(a2)/1
  [BETA] -> Cn_dr30(a,b)/2
  [ALPHA] -> Cn_dr30(a,b)/1
  [ALPHA] -> Cn_da20_lef(a2,b)/1
  [ALPHA] -> Cn_da20(a,b)/1
  [ALPHA] -> Cn(a,b,de=0)/1
  [ALPHA] -> Cn_lef(a2,b)/1
  Constant7/1 -> Cn(a,b,de=0)/3
  [DE] -> Cn(a,b,de2)/3
  [CY_tot] -> getCnt/3(CY_tot)
  getCnt/1(Cn_tot) -> [Cn_tot]
  getCnt/2(Cn_trim) -> [Cn_trim]
  getCnt/3(Cn_da) -> [Cn_da]
  getCnt/4(Cn_dr) -> [Cn_dr]
  dClp_lef(a2)/1 -> getClt/9(dClp_lef)  "dClp_lef"
  Cl_lef(a2,b)/1 -> Subtract4/1, Add8/2  "Cl_lef"
  dClbeta(a1)/1 -> getClt/10(dClbeta)  "dClbeta"
  Cl_dr30(a,b)/1 -> Subtract6/2  "Cl_dr30"
  Clr(a)/1 -> getClt/6(Clr)  "Clr"
  Subtract6/1 -> getClt/5(dCl_dr30)  "dCl_dr30"
  Clp(a)/1 -> getClt/8(Clp)  "Clp"
  Subtract4/1 -> getClt/2(dCl_lef)  "dCl_lef"
  Subtract5/1 -> getClt/3(dCl_da20)  "dCl_da20"
  Cl(a,b,de2=0)/1 -> Subtract5/1, Subtract6/1, Add8/1, Subtract4/2  "Cl(a,b,de2=0)"
  dClr_lef(a2)/1 -> getClt/7(dClr_lef)  "dClr_lef"
  Cl(a,b,de2)/1 -> getClt/1(Cl)
  Cl_da20(a,b)/1 -> Add8/3, Subtract5/2  "Cl_da20"
  Cl_da20_lef(a,b)/1 -> Add8/4  "Cl_da20_lef"
  Add8/1 -> getClt/4(dCl_da20_lef)
  [ALPHA] -> Cl(a,b,de2)/1
  [BETA] -> Cl(a,b,de2)/2
  [BETA] -> Cl_lef(a2,b)/2
  [ALPHA] -> Cl_lef(a2,b)/1
  [ALPHA] -> dClbeta(a1)/1
  [ALPHA] -> dClp_lef(a2)/1
  [ALPHA] -> Clp(a)/1
  [ALPHA] -> dClr_lef(a2)/1
  [ALPHA] -> Clr(a)/1
  [BETA] -> Cl_dr30(a,b)/2
  [ALPHA] -> Cl_dr30(a,b)/1
  [ALPHA] -> Cl_da20_lef(a,b)/1
  [BETA] -> Cl_da20_lef(a,b)/2
  [BETA] -> Cl_da20(a,b)/2
  [ALPHA] -> Cl_da20(a,b)/1
  [BETA] -> Cl(a,b,de2=0)/2
  [ALPHA] -> Cl(a,b,de2=0)/1
  Constant8/1 -> Cl(a,b,de2=0)/3
  [DE] -> Cl(a,b,de2)/3
  getClt/1(Cl_tot) -> [Cl_tot]
  getClt/2(Cl_trim) -> [Cl_trim]
  getClt/3(Cl_da) -> [Cl_da]
  getClt/4(Cl_dr) -> [Cl_dr]
  [Xcg_ref] -> getCnt/17(xcgr)
  [Xcg] -> getCnt/18(xcg)
  [r_body] -> getCnt/12(r)
  [p_body] -> getCnt/13(p)
  [DLEF] -> getCnt/14(DLEF)
  [DR] -> getCnt/15(DR)
  [DA] -> getCnt/16(DA)
  [cref] -> getCnt/19(cbar)
  [spd] -> getCnt/21(V)
  [bref] -> getCnt/20(b)
  [BETA] -> getCnt/22(beta)
  [BETA] -> getClt/18(beta)
  [spd] -> getClt/17(V)
  [r_body] -> getClt/16(r)
  [p_body] -> getClt/15(p)
  [bref] -> getClt/14(b)
  [DA] -> getClt/12(DA)
  [DLEF] -> getClt/11(DLEF)
  [DR] -> getClt/13(DR)
  [Cl_trim] -> Mux/1
  [Cm_trim] -> Mux/2
  [Cn_trim] -> Mux/3
  Mux/1 -> OUT_Clmn_trim/1
  [Cl_da] -> Mux1/1
  [Cl_dr] -> Mux1/2
  Mux1/1 -> OUT_Cln_dadr/1
  [Cn_da] -> Mux1/3
  [Cn_dr] -> Mux1/4
  [Cm_tot] -> OUT_Cmt/1
  [Cn_tot] -> OUT_Cnt/1
  [Cl_tot] -> OUT_Clt/1
  [CZ_tot] -> OUT_CZt/1
  [CX_tot] -> OUT_CXt/1
  [CY_tot] -> OUT_CYt/1

== matlab function M_DYN_AerodynamicData/getCYt ==
  data: CY input; CY_tot output; dCY_lef input; dCY_a20 input; dCY_a20_lef input; dCY_r30 input; CYr input; dCYr_lef input; CYp input; dCYp_lef input; DLEF input; DA input; DR input; b input; p input; r input; V input
function CY_tot = getCYt(CY, dCY_lef, dCY_a20, dCY_a20_lef, dCY_r30, CYr, dCYr_lef, CYp, dCYp_lef, DLEF, DA, DR, b, p, r, V)

% Detour for divide by zero
V = V + 1e-6;

CY_tot = CY ...
    + dCY_lef*(1-DLEF/25) ...
    + (dCY_a20 + dCY_a20_lef*(1-DLEF/25))*(DA/20) ...
    + dCY_r30*(DR/30) ...
    + r*b/(2*V)*(CYr+dCYr_lef*(1-DLEF/25)) ...
    + p*b/(2*V)*(CYp+dCYp_lef*(1-DLEF/25));
end

== matlab function M_DYN_AerodynamicData/getCnt ==
  data: Cn_tot output; Cn input; dCn_lef input; CY_tot input; dCn_a20 input; dCn_a20_lef input; dCn_r30 input; Cnr input; dCnr_lef input; Cnp input; dCnp_lef input; dCnbeta input; r input; p input; DLEF input; DR input; DA input; xcgr input; xcg input; cbar input; b input; V input; beta input; Cn_trim output; Cn_da output; Cn_dr output
function [Cn_tot, Cn_trim, Cn_da, Cn_dr] = getCnt(Cn, dCn_lef, CY_tot, dCn_a20, dCn_a20_lef, dCn_r30, Cnr, dCnr_lef, Cnp, dCnp_lef, dCnbeta, r, p, DLEF, DR, DA, xcgr, xcg, cbar, b, V, beta)

% Detour for divide by zero
V = V + 1e-6;

Cn_tot = Cn ...
    + dCn_lef*(1-DLEF/25) ...
    - CY_tot*(xcgr-xcg)*cbar/b ...
    + (dCn_a20 + dCn_a20_lef*(1-DLEF/25))*(DA/20) ...
    + r*b/(2*V)*(Cnr+dCnr_lef*(1-DLEF/25)) ...
    + p*b/(2*V)*(Cnp+dCnp_lef*(1-DLEF/25)) ...
    + dCn_r30*(DR/30) ...
    + dCnbeta;

Cn_trim = Cn ...
    + dCn_lef*(1-DLEF/25) ...
    - CY_tot*(xcgr-xcg)*cbar/b ...
    + r*b/(2*V)*(Cnr+dCnr_lef*(1-DLEF/25)) ...
    + p*b/(2*V)*(Cnp+dCnp_lef*(1-DLEF/25)) ...
    + dCnbeta;

Cn_da = (dCn_a20 + dCn_a20_lef*(1-DLEF/25))/20;

Cn_dr = dCn_r30/30;

== matlab function M_DYN_AerodynamicData/getClt ==
  data: Cl_tot output; Cl input; dCl_lef input; dCl_da20 input; dCl_da20_lef input; dCl_dr30 input; Clr input; dClr_lef input; Clp input; dClp_lef input; dClbeta input; DLEF input; DA input; DR input; b input; p input; r input; V input; beta input; Cl_trim output; Cl_da output; Cl_dr output
function [Cl_tot, Cl_trim, Cl_da, Cl_dr] = getClt(Cl, dCl_lef, dCl_da20,  dCl_da20_lef, dCl_dr30, Clr, dClr_lef, Clp, dClp_lef, dClbeta, DLEF, DA, DR, b, p, r, V, beta)

% Detour for divide by zero
V = V + 1e-6;

Cl_tot  = Cl + dCl_lef*(1-DLEF/25) ...
    + (dCl_da20+dCl_da20_lef*(1-DLEF/25))*(DA/20) ...
    + dCl_dr30*(DR/30) ...
    + (b/(2*V))*( (Clr+dClr_lef*(1-DLEF/25))*r + (Clp+dClp_lef*(1-DLEF/25))*p ) ...
    + dClbeta * beta;

Cl_trim = Cl + dCl_lef*(1-DLEF/25) ...
    + (b/(2*V))*( (Clr+dClr_lef*(1-DLEF/25))*r + (Clp+dClp_lef*(1-DLEF/25))*p ) ...
    + dClbeta * beta;

Cl_da  = (dCl_da20+dCl_da20_lef*(1-DLEF/25))/20;
Cl_dr  =  dCl_dr30/30;


end

== matlab function M_DYN_AerodynamicData/getCZt ==
  data: CZ input; CZ_tot output; dCZ_lef input; CZq input; CZq_lef input; DLEF input; cbar input; q input; V input
function CZ_tot = getCZt(CZ, dCZ_lef, CZq, CZq_lef, DLEF, cbar, q, V)

% Detour for divide by zero
V = V + 1e-6;

CZ_tot = CZ + dCZ_lef*(1-DLEF/25) + cbar*q/(2*V)*(CZq + CZq_lef*(1-DLEF/25));

== matlab function M_DYN_AerodynamicData/getCXt ==
  data: CX input; CX_tot output; dCX_lef input; CXq input; dCXq_lef input; DLEF input; cbar input; q input; V input
function CX_tot = getCXt(CX, dCX_lef, CXq, dCXq_lef, DLEF, cbar, q, V)

% Detour for divide by zero
V = V + 1e-4;

CX_tot = CX ...
    + dCX_lef*(1-DLEF/25) ...
    + q*cbar/(2*V)*(CXq+dCXq_lef*(1-DLEF/25));

end

== matlab function M_DYN_AerodynamicData/getCmt ==
  data: Cm input; CZ_tot input; Cm_tot output; dCm_lef input; Cmq input; dCmq_lef input; dCm input; dCm_ds input; cbar input; DLEF input; q input; V input; xcg input; xcgr input; Cm_trim output; Cm_de output
function [Cm_tot, Cm_trim, Cm_de] = getCmt(Cm, CZ_tot, dCm_lef, Cmq, dCmq_lef, dCm, dCm_ds, cbar, DLEF, q, V, xcg, xcgr)

% Detour for divide by zero
V = V + 1e-6;

Cm_tot = Cm ...
    + CZ_tot*(xcgr - xcg) ...
    + dCm_lef*(1-DLEF/25) ...
    + cbar*q/(2*V)*( Cmq + dCmq_lef*(1-DLEF/25) ) ...
    + dCm ...
    + dCm_ds;

Cm_trim = CZ_tot*(xcgr - xcg) ...
    + dCm_lef*(1-DLEF/25) ...
    + cbar*q/(2*V)*( Cmq + dCmq_lef*(1-DLEF/25) ) ...
    + dCm;

Cm_de = Cm + dCm_ds;
